simulink model "OL_HiLData"  (R2015b)
settings: Solver=FixedStepDiscrete  StartTime=0.0  StopTime=stop_time  FixedStep=step_size  RelTol=1e-3
values from neighbouring files (symbols this model uses):
  step_size = 0.1    [loadCalib.m]
  stop_time = 660    [run_test_cases.m]
undefined symbols (not defined in the file or in its folder): canChannel
libraries: canmsglib x62, canlib x29, realtime_pacer_lib x1
(part 1 of 4)
settings Model: SimulationMode=accelerator  Creator=nctzv8  LastModifiedBy=nctzv8

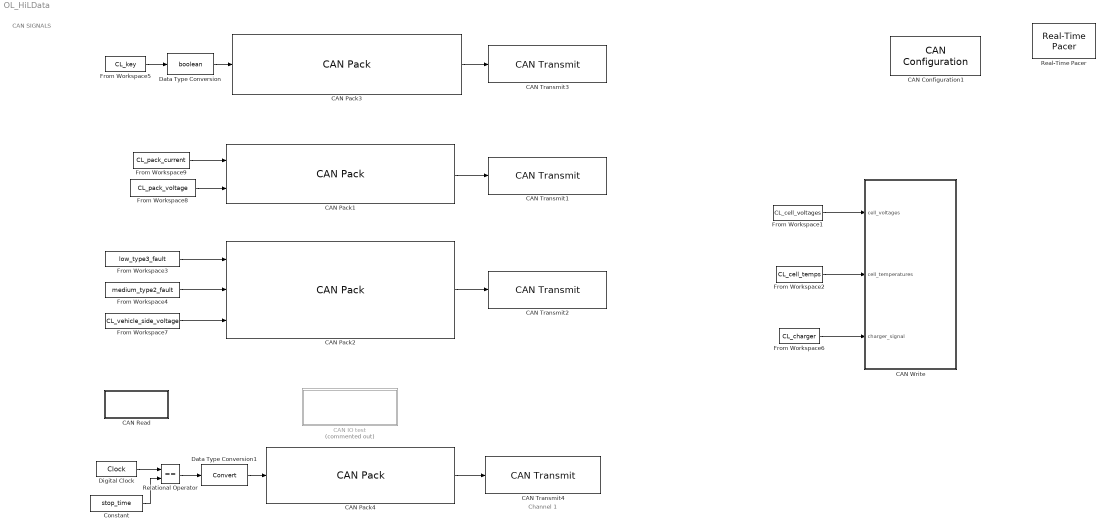
== system OL_HiLData ==
  note: CAN SIGNALS
  note: Channel 1
  CAN Configuration1 : canlib/CAN Configuration  BlockHandle=5.0001  DeviceMenu=Kvaser Leaf Light v2 1 (Channel 1)  Device=Kvaser Leaf Light v2 1 (Channel 1)  ObjConstructor=canChannel('Kvaser', 'Leaf Light v2 1', 1)  BusSpeed=500000  EnableBitParameters=off  SJW=1  TSEG1=4  TSEG2=3  NSamples=1  AckMode=Normal
  CAN IO test : Subsystem  Commented=on
  CAN Pack1 : canmsglib/CAN Pack  CANdbFile=D:\Projects\BMS\P006n\08_Work_in_progress\Repo_Sync_folder\OpenLoopDataSendCAN\BMSdb.dbc  MsgList=pack_data  MsgName=pack_data  MsgIDType=Standard (11-bit identifier)  MsgIdentifier=36  MsgLength=8  SignalInfo=pack_current$16$24$2$1$1$0$1.000000e-03$0$-200$200$#pack_voltage$40$24$2$2$1$0$1.000000e-03$0$0$200$#  NSignals=2  StartBits=str2num('[int32(16);int32(40)]')  SignalSizes=str2num('[int32(24);int32(24)]')  ByteOrders=str2num('[int32(2);int32(2)]')  DataTypes=str2num('[int32(1);int32(2)]')  MultiplexTypes=str2num('[int32(1);int32(1)]')  MultiplexValues=str2num('[double(0);double(0)]')  Factors=str2num('[double(1.000000e-03);double(1.000000e-03)]')  Offsets=str2num('[double(0);double(0)]')  Minimums=str2num('[double(-200);double(0)]')  Maximums=str2num('[double(200);double(200)]')  Remote=off
      settings: DataFormat=CANdb specified signals
  CAN Pack2 : canmsglib/CAN Pack  CANdbFile=D:\Projects\BMS\P006n\08_Work_in_progress\Repo_Sync_folder\OpenLoopDataSendCAN\BMSdb.dbc  MsgList=pack_data_2  MsgName=pack_data_2  MsgIDType=Standard (11-bit identifier)  MsgIdentifier=37  MsgLength=8  SignalInfo=low_fault$30$1$2$2$1$0$1$0$0$1$#medium_fault$31$1$2$2$1$0$1$0$0$1$#vehicle_side_voltage$16$24$2$2$1$0$1$0$0$200$#  NSignals=3  StartBits=str2num('[int32(30);int32(31);int32(16)]')  SignalSizes=str2num('[int32(1);int32(1);int32(24)]')  ByteOrders=str2num('[int32(2);int32(2);int32(2)]')  DataTypes=str2num('[int32(2);int32(2);int32(2)]')  MultiplexTypes=str2num('[int32(1);int32(1);int32(1)]')  MultiplexValues=str2num('[double(0);double(0);double(0)]')  Factors=str2num('[double(1);double(1);double(1)]')  Offsets=str2num('[double(0);double(0);double(0)]')  Minimums=str2num('[double(0);double(0);double(0)]')  Maximums=str2num('[double(1);double(1);double(200)]')  Remote=off
      settings: DataFormat=CANdb specified signals
  CAN Pack3 : canmsglib/CAN Pack  CANdbFile=D:\Projects\BMS\P006n\08_Work_in_progress\Repo_Sync_folder\OpenLoopDataSendCAN\VEHdb.dbc  MsgList=driver_info  MsgName=driver_info  MsgIDType=Standard (11-bit identifier)  MsgIdentifier=56  MsgLength=8  SignalInfo=key_status$7$1$2$2$1$0$1$0$0$1$#  NSignals=1  StartBits=str2num('[int32(7)]')  SignalSizes=str2num('[int32(1)]')  ByteOrders=str2num('[int32(2)]')  DataTypes=str2num('[int32(2)]')  MultiplexTypes=str2num('[int32(1)]')  MultiplexValues=str2num('[double(0)]')  Factors=str2num('[double(1)]')  Offsets=str2num('[double(0)]')  Minimums=str2num('[double(0)]')  Maximums=str2num('[double(1)]')  Remote=off
      settings: DataFormat=CANdb specified signals
  CAN Pack4 : canmsglib/CAN Pack  CANdbFile=D:\Projects\BMS\P006n\08_Work_in_progress\Repo_Sync_folder\OpenLoopDataSendCAN\VEHdb.dbc  MsgList=reset_cmd  MsgName=reset_cmd  MsgIDType=Standard (11-bit identifier)  MsgIdentifier=57  MsgLength=8  SignalInfo=forced_reset$7$1$2$2$1$0$1$0$0$1$#  NSignals=1  StartBits=str2num('[int32(7)]')  SignalSizes=str2num('[int32(1)]')  ByteOrders=str2num('[int32(2)]')  DataTypes=str2num('[int32(2)]')  MultiplexTypes=str2num('[int32(1)]')  MultiplexValues=str2num('[double(0)]')  Factors=str2num('[double(1)]')  Offsets=str2num('[double(0)]')  Minimums=str2num('[double(0)]')  Maximums=str2num('[double(1)]')  Remote=off
      settings: DataFormat=CANdb specified signals
  CAN Read : Subsystem
  CAN Transmit1 : canlib/CAN Transmit  BlockHandle=575.0005  DeviceMenu=Kvaser Leaf Light v2 1 (Channel 1)  Device=Kvaser Leaf Light v2 1 (Channel 1)  ObjConstructor=canChannel('Kvaser', 'Leaf Light v2 1', 1)  EnablePeriodicTransmit=off  MessagePeriod=1.000
  CAN Transmit2 : canlib/CAN Transmit  BlockHandle=576.0005  DeviceMenu=Kvaser Leaf Light v2 1 (Channel 1)  Device=Kvaser Leaf Light v2 1 (Channel 1)  ObjConstructor=canChannel('Kvaser', 'Leaf Light v2 1', 1)  EnablePeriodicTransmit=off  MessagePeriod=1.000
  CAN Transmit3 : canlib/CAN Transmit  BlockHandle=577.0005  DeviceMenu=Kvaser Leaf Light v2 1 (Channel 1)  Device=Kvaser Leaf Light v2 1 (Channel 1)  ObjConstructor=canChannel('Kvaser', 'Leaf Light v2 1', 1)  EnablePeriodicTransmit=off  MessagePeriod=1.000
  CAN Transmit4 : canlib/CAN Transmit  BlockHandle=578.0005  DeviceMenu=Kvaser Leaf Light v2 1 (Channel 1)  Device=Kvaser Leaf Light v2 1 (Channel 1)  ObjConstructor=canChannel('Kvaser', 'Leaf Light v2 1', 1)  EnablePeriodicTransmit=off  MessagePeriod=1.000
  CAN Write : Subsystem
  Constant : Constant  Value=stop_time  SampleTime=-1
  Data Type Conversion : DataTypeConversion  OutDataTypeStr=boolean
  Data Type Conversion1 : DataTypeConversion
  Digital Clock : DigitalClock  SampleTime=step_size
  From Workspace1 : FromWorkspace  VariableName=CL_cell_voltages  SampleTime=step_size
  From Workspace2 : FromWorkspace  VariableName=CL_cell_temps  SampleTime=step_size
  From Workspace3 : FromWorkspace  VariableName=low_type3_fault  SampleTime=step_size
  From Workspace4 : FromWorkspace  VariableName=medium_type2_fault  SampleTime=step_size
  From Workspace5 : FromWorkspace  VariableName=CL_key  SampleTime=step_size
  From Workspace6 : FromWorkspace  VariableName=CL_charger  SampleTime=step_size
  From Workspace7 : FromWorkspace  VariableName=CL_vehicle_side_voltage  SampleTime=step_size
  From Workspace8 : FromWorkspace  VariableName=CL_pack_voltage  SampleTime=step_size
  From Workspace9 : FromWorkspace  VariableName=CL_pack_current  SampleTime=step_size
  Real-Time Pacer : realtime_pacer_lib/Real-Time Pacer  simTimePerRealTime=1
  Relational Operator : RelationalOperator  Operator===  OutDataTypeStr=boolean
  wires:
  From Workspace1/1 -> CAN Write/1(cell_voltages)
  From Workspace2/1 -> CAN Write/2(cell_temperatures)
  From Workspace6/1 -> CAN Write/3(charger_signal)
  CAN Pack1/1 -> CAN Transmit1/1
  From Workspace9/1 -> CAN Pack1/1
  From Workspace8/1 -> CAN Pack1/2
  CAN Pack2/1 -> CAN Transmit2/1
  From Workspace7/1 -> CAN Pack2/3
  From Workspace3/1 -> CAN Pack2/1
  From Workspace4/1 -> CAN Pack2/2
  CAN Pack3/1 -> CAN Transmit3/1
  From Workspace5/1 -> Data Type Conversion/1
  Data Type Conversion/1 -> CAN Pack3/1
  CAN Pack4/1 -> CAN Transmit4/1
  Data Type Conversion1/1 -> CAN Pack4/1
  Digital Clock/1 -> Relational Operator/1
  Constant/1 -> Relational Operator/2
  Relational Operator/1 -> Data Type Conversion1/1

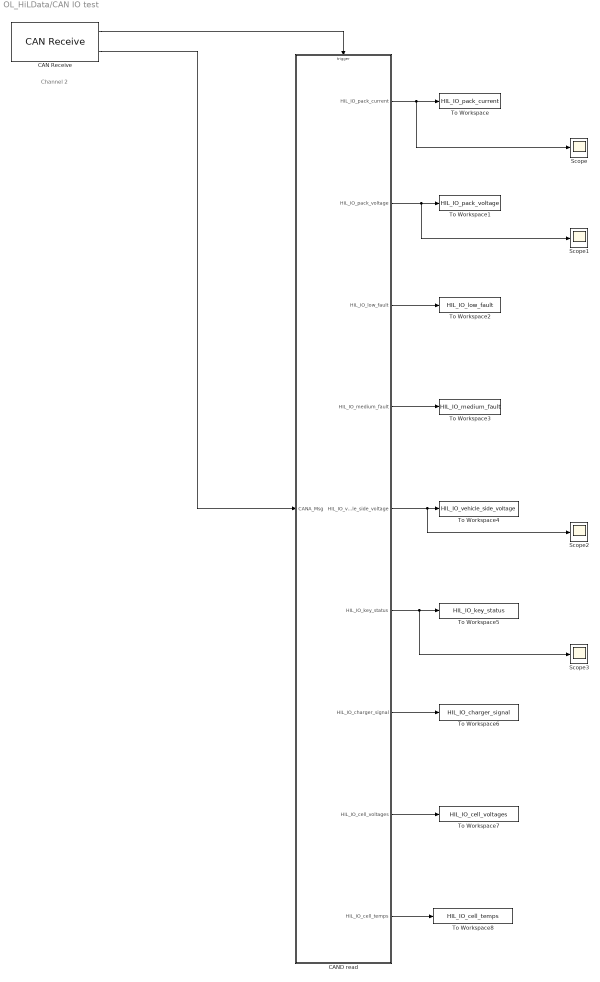
== system OL_HiLData/CAN IO test ==
  note: Channel 2
  CAN Receive : canlib/CAN Receive  BlockHandle=7.0011  DeviceMenu=Kvaser Leaf Light v2 1 (Channel 1)  Device=Kvaser Leaf Light v2 1 (Channel 1)  ObjConstructor=canChannel('Kvaser', 'Leaf Light v2 1', 1)  EnableStandardIDsFilter=off  StandardIDs=0  EnableExtendedIDsFilter=off  ExtendedIDs=0  SampleTime=step_size  MsgsPerTimestep=all  StdIDsCombo=Allow all  ExtIDsCombo=Allow all  InternalFilterUpdateStatus=on
  CAND read : Subsystem
  Scope{,1..3} (4 alike) : Scope
  To Workspace : ToWorkspace  VariableName=HIL_IO_pack_current  SaveFormat=Timeseries  SampleTime=-1
  To Workspace1 : ToWorkspace  VariableName=HIL_IO_pack_voltage  SaveFormat=Timeseries  SampleTime=-1
  To Workspace2 : ToWorkspace  VariableName=HIL_IO_low_fault  SaveFormat=Timeseries  SampleTime=-1
  To Workspace3 : ToWorkspace  VariableName=HIL_IO_medium_fault  SaveFormat=Timeseries  SampleTime=-1
  To Workspace4 : ToWorkspace  VariableName=HIL_IO_vehicle_side_voltage  SaveFormat=Timeseries  SampleTime=-1
  To Workspace5 : ToWorkspace  VariableName=HIL_IO_key_status  SaveFormat=Timeseries  SampleTime=-1
  To Workspace6 : ToWorkspace  VariableName=HIL_IO_charger_signal  SaveFormat=Timeseries  SampleTime=-1
  To Workspace7 : ToWorkspace  VariableName=HIL_IO_cell_voltages  SaveFormat=Timeseries  SampleTime=-1
  To Workspace8 : ToWorkspace  VariableName=HIL_IO_cell_temps  SaveFormat=Timeseries  SampleTime=-1
  wires:
  CAN Receive/1 -> CAND read/Trigger
  CAN Receive/2 -> CAND read/1(CANA_Msg)
  CAND read/1(HIL_IO_pack_current) -> Scope/1, To Workspace/1
  CAND read/2(HIL_IO_pack_voltage) -> Scope1/1, To Workspace1/1
  CAND read/3(HIL_IO_low_fault) -> To Workspace2/1
  CAND read/4(HIL_IO_medium_fault) -> To Workspace3/1
  CAND read/5(HIL_IO_vehicle_side_voltage) -> Scope2/1, To Workspace4/1
  CAND read/6(HIL_IO_key_status) -> Scope3/1, To Workspace5/1
  CAND read/7(HIL_IO_charger_signal) -> To Workspace6/1
  CAND read/8(HIL_IO_cell_voltages) -> To Workspace7/1
  CAND read/9(HIL_IO_cell_temps) -> To Workspace8/1

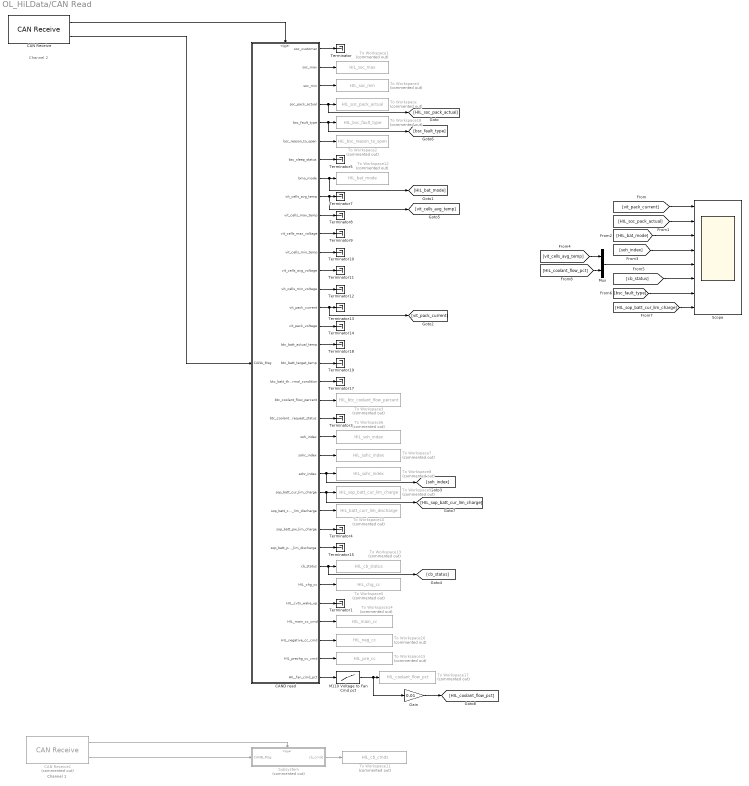
== system OL_HiLData/CAN Read ==
  note: Channel 1
  note: Channel 2
  CAN Receive : canlib/CAN Receive  BlockHandle=261.0001  DeviceMenu=Kvaser Leaf Light v2 1 (Channel 1)  Device=Kvaser Leaf Light v2 1 (Channel 1)  ObjConstructor=canChannel('Kvaser', 'Leaf Light v2 1', 1)  EnableStandardIDsFilter=off  StandardIDs=0  EnableExtendedIDsFilter=off  ExtendedIDs=0  SampleTime=step_size  MsgsPerTimestep=all  StdIDsCombo=Allow all  ExtIDsCombo=Allow all  InternalFilterUpdateStatus=on
  CAN Receive1 : canlib/CAN Receive  Commented=on  BlockHandle=262.0001  DeviceMenu=Kvaser Leaf Light v2 1 (Channel 1)  Device=Kvaser Leaf Light v2 1 (Channel 1)  ObjConstructor=canChannel('Kvaser', 'Leaf Light v2 1', 1)  EnableStandardIDsFilter=off  StandardIDs=0  EnableExtendedIDsFilter=off  ExtendedIDs=0  SampleTime=step_size  MsgsPerTimestep=all  StdIDsCombo=Allow all  ExtIDsCombo=Allow all  InternalFilterUpdateStatus=on
  CAND read : Subsystem
  Gain : Gain  Gain=0.01
  M110 Voltage to Fan Cmd pct : Lookup_n-D  NumberOfTableDimensions=1  BreakpointsForDimension1=[0 5]  Table=[0 100]  InternalRulePriority=Speed  RndMeth=Simplest  InputSameDT=on
  Mux : Mux  Inputs=2
  Scope : Scope  NumInputPorts=8
  Subsystem : Subsystem  Commented=on
  Terminator{,1,3..5,7..15,17..19} (17 alike) : Terminator
  To Workspace : ToWorkspace  Commented=on  VariableName=HIL_soc_pack_actual  SaveFormat=Timeseries  SampleTime=-1
  To Workspace1 : ToWorkspace  Commented=on  VariableName=HIL_soc_max  SaveFormat=Timeseries  SampleTime=-1
  To Workspace10 : ToWorkspace  Commented=on  VariableName=HIL_batt_curr_lim_discharge  SaveFormat=Timeseries  SampleTime=-1
  To Workspace11 : ToWorkspace  Commented=on  VariableName=HIL_cb_cmds  SaveFormat=Timeseries  SampleTime=-1
  To Workspace12 : ToWorkspace  Commented=on  VariableName=HIL_bat_mode  SaveFormat=Timeseries  SampleTime=-1
  To Workspace13 : ToWorkspace  Commented=on  VariableName=HIL_cb_status  SaveFormat=Timeseries  SampleTime=-1
  To Workspace14 : ToWorkspace  Commented=on  VariableName=HIL_main_cc  SaveFormat=Timeseries  SampleTime=-1
  To Workspace15 : ToWorkspace  Commented=on  VariableName=HIL_pre_cc  SaveFormat=Timeseries  SampleTime=-1
  To Workspace16 : ToWorkspace  Commented=on  VariableName=HIL_neg_cc  SaveFormat=Timeseries  SampleTime=-1
  To Workspace17 : ToWorkspace  Commented=on  VariableName=HIL_coolant_flow_pct  SaveFormat=Timeseries  SampleTime=-1
  To Workspace18 : ToWorkspace  Commented=on  VariableName=HIL_bsc_fault_type  SaveFormat=Timeseries  SampleTime=-1
  To Workspace2 : ToWorkspace  Commented=on  VariableName=HIL_bsc_reason_to_open  SaveFormat=Timeseries  SampleTime=-1
  To Workspace3 : ToWorkspace  Commented=on  VariableName=HIL_btc_coolant_flow_percent  SaveFormat=Timeseries  SampleTime=-1
  To Workspace4 : ToWorkspace  Commented=on  VariableName=HIL_soc_min  SaveFormat=Timeseries  SampleTime=-1
  To Workspace5 : ToWorkspace  Commented=on  VariableName=HIL_chg_cc  SaveFormat=Timeseries  SampleTime=-1
  To Workspace6 : ToWorkspace  Commented=on  VariableName=HIL_soh_index  SaveFormat=Timeseries  SampleTime=-1
  To Workspace7 : ToWorkspace  Commented=on  VariableName=HIL_sohc_index  SaveFormat=Timeseries  SampleTime=-1
  To Workspace8 : ToWorkspace  Commented=on  VariableName=HIL_sohr_index  SaveFormat=Timeseries  SampleTime=-1
  To Workspace9 : ToWorkspace  Commented=on  VariableName=HIL_sop_batt_cur_lim_charge  SaveFormat=Timeseries  SampleTime=-1
  wires:
  CAN Receive/2 -> CAND read/1(CANA_Msg)
  CAND read/1(soc_customer) -> Terminator/1
  CAND read/2(soc_max) -> To Workspace1/1
  CAND read/3(soc_min) -> To Workspace4/1
  CAND read/4(soc_pack_actual) -> [HIL_soc_pack_actual], To Workspace/1
  CAND read/5(bsc_fault_type) -> [bsc_fault_type], To Workspace18/1
  CAND read/6(bsc_reason_to_open) -> To Workspace2/1
  CAND read/7(bsc_sleep_status) -> Terminator5/1
  CAND read/8(bmo_mode) -> [HIL_bat_mode], To Workspace12/1
  CAND read/9(vit_cells_avg_temp) -> [vit_cells_avg_temp], Terminator7/1
  CAND read/10(vit_cells_max_temp) -> Terminator8/1
  CAND read/11(vit_cells_max_voltage) -> Terminator9/1
  CAND read/12(vit_cells_min_temp) -> Terminator10/1
  CAND read/13(vit_cells_avg_voltage) -> Terminator11/1
  CAND read/14(vit_cells_min_voltage) -> Terminator12/1
  CAND read/15(vit_pack_current) -> [vit_pack_current], Terminator13/1
  CAND read/16(vit_pack_voltage) -> Terminator14/1
  CAND read/17(btc_batt_actual_temp) -> Terminator18/1
  CAND read/18(btc_batt_target_temp) -> Terminator19/1
  CAND read/19(btc_batt_thermal_condition) -> Terminator17/1
  CAND read/20(btc_coolant_flow_percent) -> To Workspace3/1
  CAND read/21(btc_coolant_request_status) -> Terminator3/1
  CAND read/22(soh_index) -> To Workspace6/1
  CAND read/23(sohc_index) -> To Workspace7/1
  CAND read/24(sohr_index) -> [soh_index], To Workspace8/1
  CAND read/25(sop_batt_cur_lim_charge) -> [HIL_sop_batt_cur_lim_charge], To Workspace9/1
  CAND read/26(sop_batt_curr_lim_discharge) -> To Workspace10/1
  CAND read/27(sop_batt_pw_lim_charge) -> Terminator4/1
  CAND read/28(sop_batt_pw_lim_discharge) -> Terminator15/1
  CAND read/29(cb_status) -> [cb_status], To Workspace13/1
  CAN Receive1/1 -> Subsystem/Trigger
  CAN Receive1/2 -> Subsystem/1(CANB_Msg)
  Subsystem/1(cb_cmds) -> To Workspace11/1
  CAND read/30(HIL_chg_cc) -> To Workspace5/1
  CAN Receive/1 -> CAND read/Trigger
  CAND read/33(HIL_negative_cc_cmd) -> To Workspace16/1
  CAND read/34(HIL_prechg_cc_cmd) -> To Workspace15/1
  CAND read/32(HIL_main_cc_cmd) -> To Workspace14/1
  CAND read/31(HIL_cvtn_wake_up) -> Terminator1/1
  M110 Voltage to Fan Cmd pct/1 -> Gain/1, To Workspace17/1
  CAND read/35(HIL_fan_cmd_pct) -> M110 Voltage to Fan Cmd pct/1
  [vit_pack_current] -> Scope/1
  [HIL_soc_pack_actual] -> Scope/2
  [HIL_bat_mode] -> Scope/3
  [soh_index] -> Scope/4
  [cb_status] -> Scope/6
  [bsc_fault_type] -> Scope/7
  [HIL_sop_batt_cur_lim_charge] -> Scope/8
  Gain/1 -> [HIL_coolant_flow_pct]
  [HIL_coolant_flow_pct] -> Mux/2
  [vit_cells_avg_temp] -> Mux/1
  Mux/1 -> Scope/5

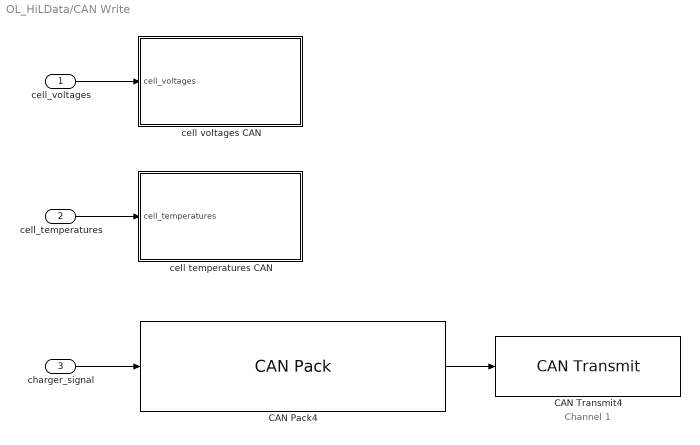
== system OL_HiLData/CAN Write ==
  note: Channel 1
  cell_voltages : Inport
  cell_temperatures : Inport  Port=2
  charger_signal : Inport  Port=3
  CAN Pack4 : canmsglib/CAN Pack  CANdbFile=D:\Projects\BMS\P006n\08_Work_in_progress\Repo_Sync_folder\OpenLoopDataSendCAN\BMSdb.dbc  MsgList=socket_charging  MsgName=socket_charging  MsgIDType=Standard (11-bit identifier)  MsgIdentifier=35  MsgLength=8  SignalInfo=charger_signal$7$1$2$2$1$0$1$0$0$1$#  NSignals=1  StartBits=str2num('[int32(7)]')  SignalSizes=str2num('[int32(1)]')  ByteOrders=str2num('[int32(2)]')  DataTypes=str2num('[int32(2)]')  MultiplexTypes=str2num('[int32(1)]')  MultiplexValues=str2num('[double(0)]')  Factors=str2num('[double(1)]')  Offsets=str2num('[double(0)]')  Minimums=str2num('[double(0)]')  Maximums=str2num('[double(1)]')  Remote=off
      settings: DataFormat=CANdb specified signals
  CAN Transmit4 : canlib/CAN Transmit  BlockHandle=584.0005  DeviceMenu=Kvaser Leaf Light v2 1 (Channel 1)  Device=Kvaser Leaf Light v2 1 (Channel 1)  ObjConstructor=canChannel('Kvaser', 'Leaf Light v2 1', 1)  EnablePeriodicTransmit=off  MessagePeriod=1.000
  cell temperatures CAN : Subsystem
  cell voltages CAN : Subsystem
  wires:
  cell_voltages/1 -> cell voltages CAN/1(cell_voltages)
  cell_temperatures/1 -> cell temperatures CAN/1(cell_temperatures)
  CAN Pack4/1 -> CAN Transmit4/1
  charger_signal/1 -> CAN Pack4/1
